simulink model "python_in_task"  (Simulink 3.00)
libraries: genlib x3, mathlib x1

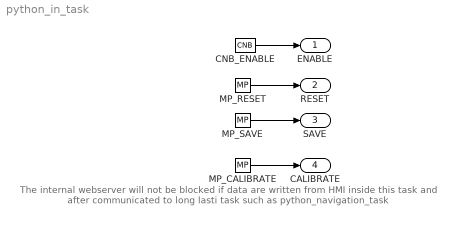
== system python_in_task ==
  note: The internal webserver will not be blocked
      | if data are written from HMI inside this task and
      | after communicated to long lasti task
      | such as python_navigation_task
  CNB_ENABLE : mathlib/CNB  YCN=on
  MP_CALIBRATE : genlib/MP  BSTATE=off  pwidth=0.001  RPTF=off
  MP_RESET : genlib/MP  BSTATE=off  pwidth=0.001  RPTF=off
  MP_SAVE : genlib/MP  BSTATE=off  pwidth=0.001  RPTF=off
  ENABLE : Outport  Port=1  OutDataTypeStr=Inherit: auto
  RESET : Outport  Port=2  OutDataTypeStr=Inherit: auto
  SAVE : Outport  Port=3  OutDataTypeStr=Inherit: auto
  CALIBRATE : Outport  Port=4  OutDataTypeStr=Inherit: auto
  wires:
  CNB_ENABLE/1 -> ENABLE/1
  MP_CALIBRATE/1 -> CALIBRATE/1
  MP_RESET/1 -> RESET/1
  MP_SAVE/1 -> SAVE/1
